simulink model "discrete"  (R2012b)
settings: Solver=VariableStepDiscrete  StartTime=0.0  StopTime=10.0  RelTol=1e-3
settings Model: Creator=stsuei  LastModifiedBy=stsuei

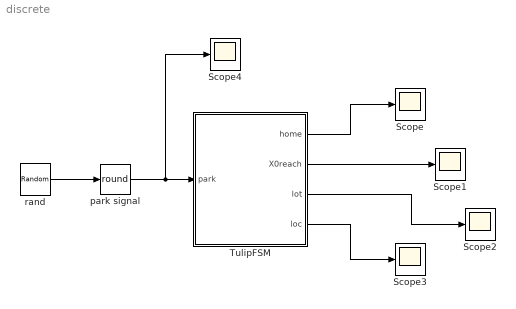
== system discrete ==
  Scope{,1..4} (5 alike) : Scope
      Scope2 settings: SaveName=ScopeData2
      Scope3 settings: SaveName=ScopeData3
      Scope4 settings: SaveName=ScopeData4
  TulipFSM : Stateflow chart  TreatAsAtomicUnit=on
  park signal : Rounding  Operator=round
  rand : UniformRandomNumber  Minimum=0  SampleTime=1
  wires:
  TulipFSM/4(loc) -> Scope3/1
  TulipFSM/1(home) -> Scope/1
  TulipFSM/2(X0reach) -> Scope1/1
  TulipFSM/3(lot) -> Scope2/1
  park signal/1 -> Scope4/1, TulipFSM/1(park)
  rand/1 -> park signal/1

== stateflow chart discrete/TulipFSM ==
  settings: updateMethod=DISCRETE  sampleTime=1  stateMachineType=MEALY_MACHINE
  state s0
  state s1
  state s2
  state s3
  state s4
  state s5
  state s6
  state s7
  state s8
  state s9
  state s10
  state s11
  state s12
  state s13
  state sSinit
  s0 -> s11 [order 2] : [(park==0)]{home=0;X0reach=0;lot=0;loc=1;}
  s0 -> s10 [order 1] : [(park==1)]{home=0;X0reach=0;lot=0;loc=1;}
  s3 -> s0 [order 1] : [(park==1)]{home=0;X0reach=1;lot=0;loc=4;}
  s2 -> s0 [order 1] : [(park==1)]{home=0;X0reach=1;lot=0;loc=4;}
  s1 -> s11 [order 2] : [(park==0)]{home=0;X0reach=0;lot=0;loc=1;}
  s1 -> s10 [order 1] : [(park==1)]{home=0;X0reach=0;lot=0;loc=1;}
  s3 -> s1 [order 2] : [(park==0)]{home=0;X0reach=1;lot=0;loc=4;}
  s2 -> s1 [order 2] : [(park==0)]{home=0;X0reach=1;lot=0;loc=4;}
  s5 -> s2 [order 1] : [(park==1)]{home=0;X0reach=0;lot=1;loc=5;}
  s4 -> s2 [order 1] : [(park==1)]{home=0;X0reach=0;lot=1;loc=5;}
  s5 -> s3 [order 2] : [(park==0)]{home=0;X0reach=0;lot=1;loc=5;}
  s4 -> s3 [order 2] : [(park==0)]{home=0;X0reach=0;lot=1;loc=5;}
  s7 -> s4 [order 1] : [(park==1)]{home=0;X0reach=0;lot=0;loc=4;}
  s6 -> s4 [order 1] : [(park==1)]{home=0;X0reach=0;lot=0;loc=4;}
  s7 -> s5 [order 2] : [(park==0)]{home=0;X0reach=0;lot=0;loc=4;}
  s6 -> s5 [order 2] : [(park==0)]{home=0;X0reach=0;lot=0;loc=4;}
  s9 -> s6 [order 1] : [(park==1)]{home=0;X0reach=0;lot=0;loc=1;}
  s8 -> s6 [order 1] : [(park==1)]{home=0;X0reach=0;lot=0;loc=1;}
  s9 -> s7 [order 2] : [(park==0)]{home=0;X0reach=0;lot=0;loc=1;}
  s8 -> s7 [order 2] : [(park==0)]{home=0;X0reach=0;lot=0;loc=1;}
  s11 -> s8 [order 1] : [(park==1)]{home=1;X0reach=0;lot=0;loc=0;}
  s10 -> s8 [order 1] : [(park==1)]{home=1;X0reach=0;lot=0;loc=0;}
  s11 -> s9 [order 2] : [(park==0)]{home=1;X0reach=0;lot=0;loc=0;}
  s10 -> s9 [order 2] : [(park==0)]{home=1;X0reach=0;lot=0;loc=0;}
  s13 -> s10 [order 1] : [(park==1)]{home=0;X0reach=0;lot=0;loc=1;}
  s12 -> s10 [order 1] : [(park==1)]{home=0;X0reach=0;lot=0;loc=1;}
  s13 -> s11 [order 2] : [(park==0)]{home=0;X0reach=0;lot=0;loc=1;}
  s12 -> s11 [order 2] : [(park==0)]{home=0;X0reach=0;lot=0;loc=1;}
  sSinit -> s12 [order 1] : [(park==0)]{home=1;X0reach=1;lot=0;loc=0;}
  sSinit -> s13 [order 2] : [(park==1)]{home=1;X0reach=1;lot=0;loc=0;}
  (default) -> sSinit
  data: park input double; home output double; X0reach output double; lot output double; loc output double
